simulink model "Example3_Calibrating_The_AR_Drone"  (R2016a)
settings: configuration reference "AR_Drone_ConfigSet" (kept outside this file)
undefined symbols (not defined in the file or in its folder): Accel_Calib_Gain, Accel_Calib_Offset, DiscIntNeverNeededParam, Mag_Calib_Gain_Vector, Mag_Calib_Offset_Vector
libraries: simulink x5, vrlib x2, AR_Drone_2_Library x1
(part 2 of 2)

== matlab function Example3_Calibrating_The_AR_Drone/Euler Angles/Compute Euler Angles/Kalman Filter Roll ==
  data: estimated_state output; ctrl_input_gyro input; measurement_angle input
function estimated_state  = fcn( ctrl_input_gyro, measurement_angle)

persistent prev_state
if isempty(prev_state)
    prev_state = [0;0];
end
persistent covariance_correction_prev
if isempty(covariance_correction_prev)
    covariance_correction_prev = eye(2);
end

%-------------------------------
%-------------------------------
%---- Predict Stage ------------
%-------------------------------
%-------------------------------
% pix_value = 5;
Ts = 1/400;
%Process Noise
p_var =0.01;
Q = [p_var^2     0         
      0         p_var^2];

%A matrix
A =  [1   -Ts 
      0   1];

%odutput these values with a unit delay (for algebraic loop), apply initial conditions
state_prediction = A*prev_state + [Ts 0; 0 0]*[ctrl_input_gyro; 0 ];
covariance_prediction = A*covariance_correction_prev*A' + Q;

%-------------------------------
%-------------------------------
%---- Estimate Stage -----------
%-------------------------------
%-------------------------------

%H matrix
H = [1 0];

%Measurement noise from accelerometer angle measurement
m_var = 0.5;
R = [m_var^2 ];

%Measurement Z
Z = [measurement_angle];

%Compute Kalman Gain
Kalman_Gain = covariance_prediction*H'*inv(H*covariance_prediction*H'+R); %2x2 matrix

%compute state space correction based on measurement
state_correction = state_prediction + Kalman_Gain*(Z - H*state_prediction); %4x1 vector of states

%compute covariance correction
covariance_correction = (eye(2) - Kalman_Gain*H)*covariance_prediction; %2x2 covariance matrix

%save the found values for the next sample
estimated_state = state_correction (1);
prev_state = state_correction;
covariance_correction_prev = covariance_correction;
 end

== matlab function Example3_Calibrating_The_AR_Drone/Euler Angles/Compute Euler Angles/Kalman Filter Pitch ==
  data: estimated_state output; ctrl_input_gyro input; measurement_angle input
function estimated_state  = fcn(ctrl_input_gyro, measurement_angle)


persistent prev_state
if isempty(prev_state)
    prev_state = [0;0];
end
persistent covariance_correction_prev
if isempty(covariance_correction_prev)
    covariance_correction_prev = eye(2);
end


%-------------------------------
%-------------------------------
%---- Predict Stage ------------
%-------------------------------
%-------------------------------
% pix_value = 5;
Ts = 1/400;
%Process Noise
p_var =0.01;
Q = [p_var^2     0         
      0         p_var^2];

%A matrix
A =  [1   -Ts 
      0   1];

%odutput these values with a unit delay (for algebraic loop), apply initial conditions
state_prediction = A*prev_state + [Ts 0; 0 0]*[ctrl_input_gyro; 0 ];
covariance_prediction = A*covariance_correction_prev*A' + Q;

%-------------------------------
%-------------------------------
%---- Estimate Stage -----------
%-------------------------------
%-------------------------------

%H matrix
H = [1 0];

%Measurement noise from accelerometer angle measurement
m_var = 1;
%     m_var_r = 1;

R = [m_var^2 ];

%Measurement Z
Z = [measurement_angle];

%Compute Kalman Gain
Kalman_Gain = covariance_prediction*H'*inv(H*covariance_prediction*H'+R); %2x2 matrix

%compute state space correction based on measurement
state_correction = state_prediction + Kalman_Gain*(Z - H*state_prediction); %4x1 vector of states

%compute covariance correction
covariance_correction = (eye(2) - Kalman_Gain*H)*covariance_prediction; %2x2 covariance matrix

%save the found values for the next sample
estimated_state = state_correction (1);
prev_state = state_correction;
covariance_correction_prev = covariance_correction;
end
